simulink library "fdclib1"  (Simulink 3.00)
undefined symbols (not defined in the file): GM1
libraries: fdclib1 x4
settings Model: LastModifiedBy=Dutchroll

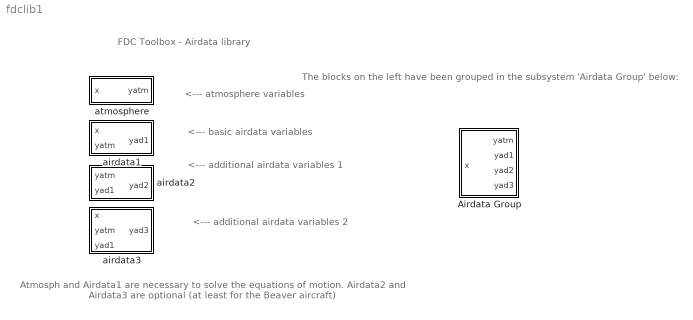
== system fdclib1 ==
  note: The blocks on the left have been grouped
      | in the subsystem 'Airdata Group' below:
  note: <--- additional airdata variables 2
  note: <--- additional airdata variables 1
  note: <--- atmosphere variables
  note: <--- basic airdata variables
  note: FDC Toolbox - Airdata library
  note: Atmosph and Airdata1 are necessary to solve the
      | equations of motion. Airdata2 and Airdata3 are
      | optional (at least for the Beaver aircraft)
  Airdata Group : Subsystem
  airdata1 : Subsystem
      mask Type: Airdata1
      mask Description: Basic airdata variables
      mask Help: eval('browse airdata1')
      mask Display: disp('Airdata1')
  airdata2 : Subsystem
      mask Type: Airdata2
      mask Description: More airdata variables
      mask Help: eval('browse airdata2')
      mask Display: disp('Airdata2')
  airdata3 : Subsystem  mask(Airdata3){cbar=GM1(1)}
      mask prompts: cbar "Mean aerodynamic chord [m]:"
      mask help: More airdata variables
      mask Help: eval('browse airdata3')
      mask Display: disp('Airdata3')
  atmosphere : Subsystem
      mask Type: Atmosph
      mask Description: Atmosphere variables
      mask Help: eval('browse atmosph')
      mask Display: disp('Atmosph')

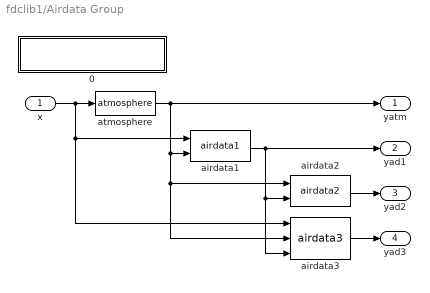
== system fdclib1/Airdata Group ==
  x : Inport  Port=1  PortWidth=-1  SampleTime=-1  DataType=auto
      settings: SignalType=auto
  0 : Subsystem
      settings: OpenFcn=browse adgrp
      mask Display: disp('AIRDATA GROUP (level 3)\nM.O. Rauw')
  airdata1 : fdclib1/airdata1
  airdata2 : fdclib1/airdata2
  airdata3 : fdclib1/airdata3  cbar=GM1(1)
  atmosphere : fdclib1/atmosphere
  yatm : Outport  Port=1
  yad1 : Outport  Port=2
  yad2 : Outport  Port=3
  yad3 : Outport  Port=4
  wires:
  airdata2/1 -> yad2/1
  airdata3/1 -> yad3/1
  atmosphere/1 -> yatm/1, airdata1/2, airdata2/1, airdata3/2
  airdata1/1 -> yad1/1, airdata2/2, airdata3/3
  x/1 -> atmosphere/1, airdata1/1, airdata3/1

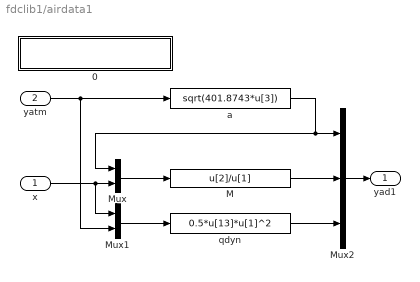
== system fdclib1/airdata1 ==
  x : Inport  Port=1  PortWidth=-1  SampleTime=-1  DataType=auto
      settings: SignalType=auto
  yatm : Inport  Port=2  PortWidth=-1  SampleTime=-1  DataType=auto
      settings: SignalType=auto
  0 : Subsystem
      settings: OpenFcn=browse airdata1
      mask Display: disp('AIRDATA1\nM.O. Rauw, March 2003')
  M : Fcn  Expr=u[2]/u[1]
  Mux : Mux  Inputs=[1 12]
      settings: DisplayOption=none
  Mux1 : Mux  Inputs=[12 5]
      settings: DisplayOption=none
  Mux2 : Mux  Inputs=3
      settings: DisplayOption=none
  a : Fcn  Expr=sqrt(401.8743*u[3])
  qdyn : Fcn  Expr=0.5*u[13]*u[1]^2
  yad1 : Outport  Port=1
  wires:
  Mux2/1 -> yad1/1
  qdyn/1 -> Mux2/3
  a/1 -> Mux/1, Mux2/1
  M/1 -> Mux2/2
  Mux1/1 -> qdyn/1
  Mux/1 -> M/1
  yatm/1 -> a/1, Mux1/2
  x/1 -> Mux/2, Mux1/1

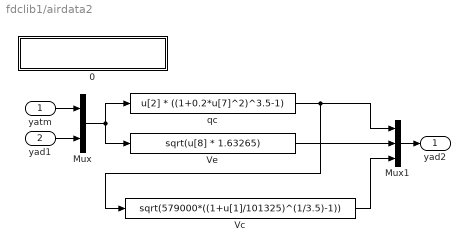
== system fdclib1/airdata2 ==
  yatm : Inport  Port=1  PortWidth=-1  SampleTime=-1  DataType=auto
      settings: SignalType=auto
  yad1 : Inport  Port=2  PortWidth=-1  SampleTime=-1  DataType=auto
      settings: SignalType=auto
  0 : Subsystem
      settings: OpenFcn=browse airdata2
      mask Display: disp('AIRDATA2\nM.O. Rauw, March 2003')
  Mux : Mux  Inputs=[5 3]
      settings: DisplayOption=none
  Mux1 : Mux  Inputs=3
      settings: DisplayOption=none
  Vc : Fcn  Expr=sqrt(579000*((1+u[1]/101325)^(1/3.5)-1))
  Ve : Fcn  Expr=sqrt(u[8] * 1.63265)
  qc : Fcn  Expr=u[2] * ((1+0.2*u[7]^2)^3.5-1)
  yad2 : Outport  Port=1
  wires:
  Mux/1 -> qc/1, Ve/1
  Ve/1 -> Mux1/2
  Vc/1 -> Mux1/3
  qc/1 -> Vc/1, Mux1/1
  Mux1/1 -> yad2/1
  yad1/1 -> Mux/2
  yatm/1 -> Mux/1

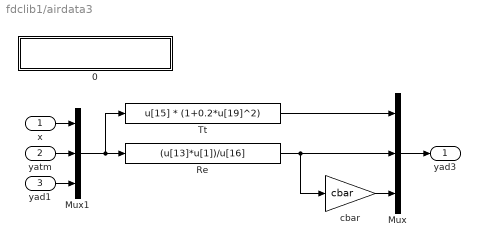
== system fdclib1/airdata3 ==
  x : Inport  Port=1  PortWidth=-1  SampleTime=-1  DataType=auto
      settings: SignalType=auto
  yatm : Inport  Port=2  PortWidth=-1  SampleTime=-1  DataType=auto
      settings: SignalType=auto
  yad1 : Inport  Port=3  PortWidth=-1  SampleTime=-1  DataType=auto
      settings: SignalType=auto
  0 : Subsystem
      settings: OpenFcn=browse airdata3
      mask Display: disp('AIRDATA3\nM.O. Rauw, March 2003')
  Mux : Mux  Inputs=3
      settings: DisplayOption=none
  Mux1 : Mux  Inputs=[12 5 3]
      settings: DisplayOption=none
  Re : Fcn  Expr=(u[13]*u[1])/u[16]
  Tt : Fcn  Expr=u[15] * (1+0.2*u[19]^2)
  cbar : Gain  Gain=cbar  SaturateOnIntegerOverflow=on
  yad3 : Outport  Port=1
  wires:
  Re/1 -> Mux/2, cbar/1
  Mux1/1 -> Re/1, Tt/1
  Mux/1 -> yad3/1
  Tt/1 -> Mux/1
  cbar/1 -> Mux/3
  x/1 -> Mux1/1
  yatm/1 -> Mux1/2
  yad1/1 -> Mux1/3

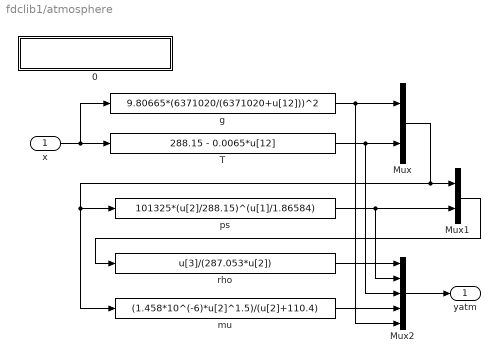
== system fdclib1/atmosphere ==
  x : Inport  Port=1  PortWidth=-1  SampleTime=-1  DataType=auto
      settings: SignalType=auto
  0 : Subsystem
      settings: OpenFcn=browse atmosph
      mask Display: disp('ATMOSPH\nM.O. Rauw, March 2003')
  Mux : Mux  Inputs=2
      settings: DisplayOption=none
  Mux1 : Mux  Inputs=[2 1]
      settings: DisplayOption=none
  Mux2 : Mux  Inputs=5
      settings: DisplayOption=none
  T : Fcn  Expr=288.15 - 0.0065*u[12]
  g : Fcn  Expr=9.80665*(6371020/(6371020+u[12]))^2
  mu : Fcn  Expr=(1.458*10^(-6)*u[2]^1.5)/(u[2]+110.4)
  ps : Fcn  Expr=101325*(u[2]/288.15)^(u[1]/1.86584)
  rho : Fcn  Expr=u[3]/(287.053*u[2])
  yatm : Outport  Port=1
  wires:
  x/1 -> T/1, g/1
  Mux/1 -> Mux1/1, mu/1, ps/1
  ps/1 -> Mux1/2, Mux2/2
  T/1 -> Mux/2, Mux2/3
  g/1 -> Mux/1, Mux2/5
  rho/1 -> Mux2/1
  Mux1/1 -> rho/1
  Mux2/1 -> yatm/1
  mu/1 -> Mux2/4

== system fdclib1/Airdata Group/0 ==

== system fdclib1/airdata1/0 ==

== system fdclib1/airdata2/0 ==

== system fdclib1/airdata3/0 ==

== system fdclib1/atmosphere/0 ==
